simulink model "control"  (R2019b)
settings: Solver=VariableStepAuto  StartTime=0.0  StopTime=10.0  RelTol=1e-3
libraries: fuzblock x1
settings Model: Creator=Laura  LastModifiedBy=Laura

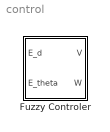
== system control ==
  Fuzzy Controler : Subsystem

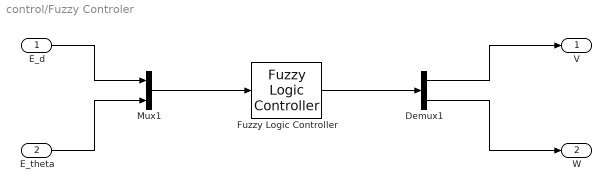
== system control/Fuzzy Controler ==
  "E_d " : Inport
  "E_theta " : Inport  Port=2
  Demux1 : Demux  Outputs=2
  Fuzzy Logic Controller : fuzblock/Fuzzy Logic  Controller  FIS='controlBorroso.fis'  OutputSampleNumber=101  DataType=double  FuzzifiedInputs=off  RuleFiringStrengths=off  RuleOutputs=off  AggregatedOutputs=off  SimulateUsing=Interpreted execution  OutOfRangeInputValueMessage=warning  NoRuleFiredMessage=warning  EmptyOutputFuzzySetMessage=warning
  Mux1 : Mux  Inputs=2
  V : Outport
  W : Outport  Port=2
  wires:
  Fuzzy Logic Controller/1 -> Demux1/1
  "E_theta "/1 -> Mux1/2
  Demux1/2 -> W/1
  Demux1/1 -> V/1
  "E_d "/1 -> Mux1/1
  Mux1/1 -> Fuzzy Logic Controller/1
